simulink model "FullESCtest"  (R2024b)
settings: Solver=VariableStepAuto  StartTime=0.0  StopTime=400  RelTol=1e-3
libraries: slctrl_adaptive x3, slpidlib x1
settings Model: Creator=Marij  LastModifiedBy=marijn
settings OptimizationCC: UseDivisionForNetSlopeComputation=on

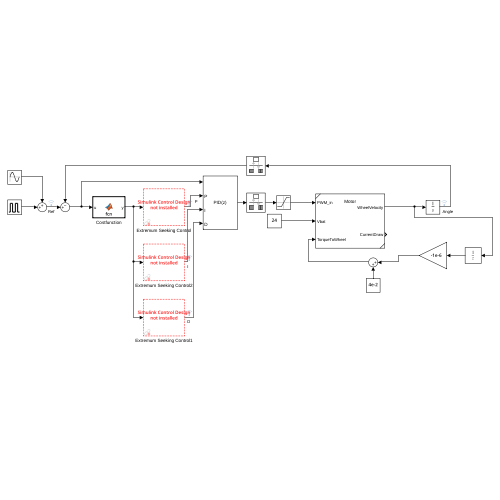
[thumbnail: Simulink's stored preview of the top-level diagram]
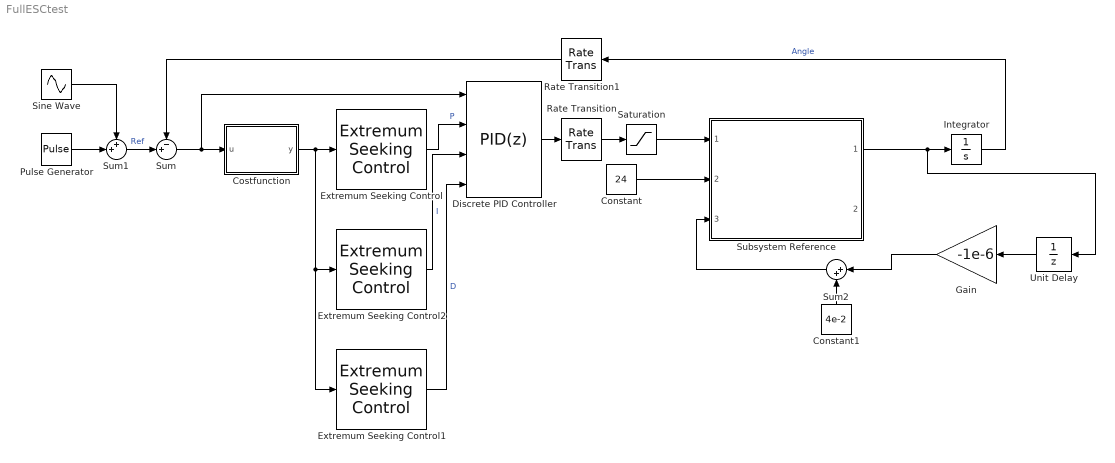
== system FullESCtest ==
  Constant : Constant  Value=24
  Constant1 : Constant  Value=4e-2
  Costfunction : MATLAB Function  TreatAsAtomicUnit=on
  Discrete PID Controller : slpidlib/PID Controller  Controller=PID  Form=Parallel  TimeDomain=Discrete-time  UseExternalTs=off  SampleTime=0.01  IntegratorMethod=Forward Euler  FilterMethod=Forward Euler  ControllerParametersSource=external  P=1  I=1  UseKiTs=off  D=0  UseExternalDerivativeSource=off  N=100  UseFilter=off  TunerSelectOption=Transfer Function Based (PID Tuner App)  InitialConditionSource=internal  InitialConditionForIntegrator=0  InitialConditionForFilter=0  DifferentiatorICPrevScaledInput=0  ExternalReset=none  TrackingMode=off  Kt=1  LimitOutput=off  SatLimitsSource=internal  UpperSaturationLimit=inf  LowerSaturationLimit=-inf  LinearizeAsGain=off  AntiWindupMode=none  Kb=1  LimitIntegrator=off  UpperIntegratorSaturationLimit=inf  LowerIntegratorSaturationLimit=-inf  POutMin=[]  POutMax=[]  IOutMin=[]  IOutMax=[]  DOutMin=[]  DOutMax=[]  NOutMin=[]  NOutMax=[]  SumOutMin=[]  SumOutMax=[]  SaturationOutMin=[]  SaturationOutMax=[]  PParamMin=[]  PParamMax=[]  IParamMin=[]  IParamMax=[]  DParamMin=[]  DParamMax=[]  NParamMin=[]  NParamMax=[]  KbParamMin=[]  KbParamMax=[]  KtParamMin=[]  KtParamMax=[]  KbOutMin=[]  KbOutMax=[]  KtOutMin=[]  KtOutMax=[]  IntegratorOutMin=[]  IntegratorOutMax=[]  FilterOutMin=[]  FilterOutMax=[]  SumI1OutMin=[]  SumI1OutMax=[]  SumI2OutMin=[]  SumI2OutMax=[]  SumI3OutMin=[]  SumI3OutMax=[]  SumI4OutMin=[]  SumI4OutMax=[]  SumDOutMin=[]  SumDOutMax=[]  DifferentiatorOutMin=[]  DifferentiatorOutMax=[]  FilterDiffOutCoefMin=[]  FilterDiffOutCoefMax=[]  ReciprocalOutMin=[]  ReciprocalOutMax=[]  SumDenOutMin=[]  SumDenOutMax=[]  SumNumOutMin=[]  SumNumOutMax=[]  DivideOutMin=[]  DivideOutMax=[]  UdiffTsProdOutMin=[]  UdiffTsProdOutMax=[]  NTsProdOutMin=[]  NTsProdOutMax=[]  UintegralTsProdOutMin=[]  UintegralTsProdOutMax=[]  UngainTsProdOutMin=[]  UngainTsProdOutMax=[]  ClampingZeroOutDataTypeStr=Inherit: Inherit via back propagation  ClampingZeroOutMin=[]  ClampingZeroOutMax=[]  FilterDenConstantOutDataTypeStr=Inherit: Inherit via back propagation  FilterDenConstantOutMin=[]  FilterDenConstantOutMax=[]  PCopyOutDataTypeStr=Inherit: Inherit via back propagation  PCopyOutMin=[]  PCopyOutMax=[]  NCopyOutDataTypeStr=Inherit: Inherit via back propagation  NCopyOutMin=[]  NCopyOutMax=[]  IntegratorContinuousStateAttributes=''  IntegratorStateMustResolveToSignalObject=off  IntegratorRTWStateStorageClass=Auto  FilterContinuousStateAttributes=''  FilterStateMustResolveToSignalObject=off  FilterRTWStateStorageClass=Auto  ParallelPVariant=ExternalParameters  IdealPVariant=Disabled  IVariant=ExternalParameters  DVariant=ExternalParameters  IntegratorVariant=Discrete  SatVariant=Disabled  AWVariant=Passthrough  PCopyVariant=Disabled  TRVariant=Disabled  FdbkBlocksVariant=Forward  IdealPFdbkVariant=Disabled  SatFdbkVariant=Disabled  DerivativeFilterVariant=Differentiator  NVariant=Passthrough  NCopyVariant=Disabled_SignalSpec  FilterICVariant=InternalICsDifferentiator  IntegratorICVariant=InternalICs  ExternalResetVariant=Disabled  TRSumVariant=Passthrough  SumFdbkVariant=Disabled  SumVariant=Sum_PID  TsampFilterVariant=InternalTs  TsampNgainVariant=Passthrough  TsampIntegralVariant=Disabled_SignalSpec  ExternalSaturationOutDataTypeStr=Inherit: Same as second input  DerivativeSourceVariant=ErrorSignal  PreIntVariant=InternalPreInt
      settings: LibrarySourceBlock=simulink/Discrete/Discrete PID Controller
  Extremum Seeking Control : slctrl_adaptive/Extremum Seeking Control  timeDomainStatus=Discrete time  SampleTime=0.01  IntegratorMethods=Trapezoidal  paramCount=1  initialVal=0.001  omega=1  gain=3e-3  demodAmp=1  demodPhase=0  modAmp=1e-5  modPhase=0  highPassEnable=off  highPassCutoff=0.5  lowPassEnable=on  lowPassCutoff=1.0  estimatedVarOn=off  HPFFreq=-0.99501  LPFFreq=-0.99005  SampleTimeVar=0.01
      settings: LibrarySourceBlock=slctrlblks/Adaptive Control/Extremum Seeking Control
  Extremum Seeking Control1 : slctrl_adaptive/Extremum Seeking Control  timeDomainStatus=Discrete time  SampleTime=0.01  IntegratorMethods=Trapezoidal  paramCount=1  initialVal=0.05  omega=1.2  gain=5e-5  demodAmp=1  demodPhase=0  modAmp=0.0005  modPhase=0  highPassEnable=on  highPassCutoff=0.1  lowPassEnable=on  lowPassCutoff=1  estimatedVarOn=off  HPFFreq=-0.999  LPFFreq=-0.99005  SampleTimeVar=0.01
      settings: LibrarySourceBlock=slctrlblks/Adaptive Control/Extremum Seeking Control
  Extremum Seeking Control2 : slctrl_adaptive/Extremum Seeking Control  timeDomainStatus=Discrete time  SampleTime=0.01  IntegratorMethods=Trapezoidal  paramCount=1  initialVal=5e-3  omega=1.4  gain=5e-5  demodAmp=1  demodPhase=0  modAmp=5e-5  modPhase=0  highPassEnable=on  highPassCutoff=0.1  lowPassEnable=on  lowPassCutoff=1  estimatedVarOn=off  HPFFreq=-0.999  LPFFreq=-0.99005  SampleTimeVar=0.01
      settings: LibrarySourceBlock=slctrlblks/Adaptive Control/Extremum Seeking Control
  Gain : Gain  Gain=-1e-6
  Integrator : Integrator
  Pulse Generator : DiscretePulseGenerator  PulseType=Time based  Period=10  PulseWidth=50  PhaseDelay=5
  Rate Transition : RateTransition  OutPortSampleTime=1e-3
  Rate Transition1 : RateTransition  OutPortSampleTime=1e-2
  Saturation : Saturate  UpperLimit=1  LowerLimit=-1
  Sine Wave : Sin  Frequency=0.5  SampleTime=0
  Subsystem Reference : Subsystem  ReferencedSubsystem=Motor
  Sum : Sum  Inputs=-+|
  Sum1 : Sum  Inputs=++|
  Sum2 : Sum  Inputs=|++
  Unit Delay : UnitDelay  SampleTime=-1  HasFrameUpgradeWarning=on
  wires:
  Constant/1 -> Subsystem Reference/2
  Sum/1 -> Discrete PID Controller/1, Costfunction/1(u)
  Subsystem Reference/1 -> Unit Delay/1, Integrator/1
  Costfunction/1(y) -> Extremum Seeking Control2/1, Extremum Seeking Control1/1, Extremum Seeking Control/1
  Discrete PID Controller/1 -> Rate Transition/1
  Integrator/1 -> Rate Transition1/1  "Angle"
  Unit Delay/1 -> Gain/1
  Extremum Seeking Control/1 -> Discrete PID Controller/2  "P"
  Extremum Seeking Control1/1 -> Discrete PID Controller/4  "D"
  Rate Transition/1 -> Saturation/1
  Rate Transition1/1 -> Sum/1
  Saturation/1 -> Subsystem Reference/1
  Sum1/1 -> Sum/2  "Ref"
  Pulse Generator/1 -> Sum1/2
  Sine Wave/1 -> Sum1/1
  Gain/1 -> Sum2/1
  Sum2/1 -> Subsystem Reference/3
  Constant1/1 -> Sum2/2
  Extremum Seeking Control2/1 -> Discrete PID Controller/3  "I"

== matlab function FullESCtest/Costfunction ==
  data: u input; y output
function y = fcn(u)
% y = abs(u);
% y = u^2;
y = abs(u^7);
